simulink model "Ejemplo_5"  (R2013a)
settings: Solver=ode45  StartTime=0.0  StopTime=100  RelTol=1e-3
settings Model: Creator=Miguel  LastModifiedBy=Miguel

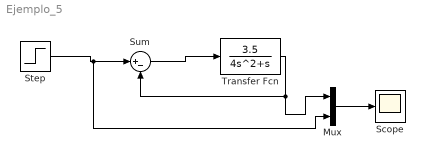
== system Ejemplo_5 ==
  Mux : Mux  Inputs=2
  Scope : Scope
      settings: TickLabels=on  ShowLegends=on
  Step : Step  SampleTime=0
  Sum : Sum  Inputs=|+-
  Transfer Fcn : TransferFcn  Numerator=[3.5]  Denominator=[4 1 0]
  wires:
  Transfer Fcn/1 -> Sum/2, Mux/1
  Mux/1 -> Scope/1
  Sum/1 -> Transfer Fcn/1
  Step/1 -> Mux/2, Sum/1
